simulink model "spring_calibration"  (R2016b)
settings: Solver=VariableStepAuto  StartTime=0.0  StopTime=3  RelTol=1e-3  EnableMultiTasking=on
values from neighbouring files (symbols this model uses):
  m = force(i)    [calibration.m]
  max_force = []    [calibration.m]
libraries: nesl_utility x4, fl_lib x4
settings Model: Creator=joachimdenil  LastModifiedBy=jdenil
settings DataIOCC: SaveFormat=Array
settings OptimizationCC: LifeSpan=inf
settings DebuggingCC: SFUnexpectedBacktrackingDiag=warning  SFNoUnconditionalDefaultTransitionDiag=warning  SFExecutionAtInitializationDiag=none
settings GRTTargetCC: TargetLangStandard=C89/C90 (ANSI)  GeneratePreprocessorConditionals=Disable all
settings ConfigComp: CovMetricSettings=dw  CovHtmlReporting=on  CovSaveCumulativeToWorkspaceVar=on  CovSaveSingleToWorkspaceVar=on  CovExternalEMLEnable=off

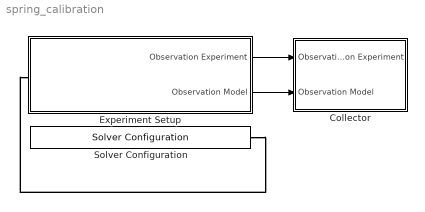
== system spring_calibration ==
  Collector : Subsystem  TreatAsAtomicUnit=on
  Experiment Setup : Subsystem
  Solver Configuration : nesl_utility/Solver Configuration  PhysicalDomain=network_engine_domain  SubClassName=solver  LeftPortType=input  RightPortType=generic  Accelerate=off  Tones=[]  Harmonics=[]  SimulateNoise=off  Profile=off  UseLocalSampling=off  EnableSwitchedLinearOptims=on  FrequencyDomain=off  UseCCode=off  RelTol=0.001  AbsTol=1e-06  MinStep=1e-09  ToWorkspace=off  RevertToSquareIcSolve=off  NumHomotopyIterations=100  PhasorMode=off  PhasorModeNumHarmonics=1  OverrideAbsTol=off  DoDC=off  ResidualTolerance=1e-09  UseLocalSolver=off  LocalSolverChoice=NE_BACKWARD_EULER_ADVANCER  LocalSolverSampleTime=0.001  DoFixedCost=off  MaxNonlinIter=3  MaxModeIter=2  LinearAlgebra=Sparse  DelaysMemoryBudget=1024  AutomaticFiltering=on  FilteringTimeConstant=0.001
  wires:
  Experiment Setup/1(Observation Experiment) -> Collector/1(Observation Experiment)
  Experiment Setup/2(Observation Model) -> Collector/2(Observation Model)
  connections:
  Solver Configuration/RConn1 -- Experiment Setup/LConn1

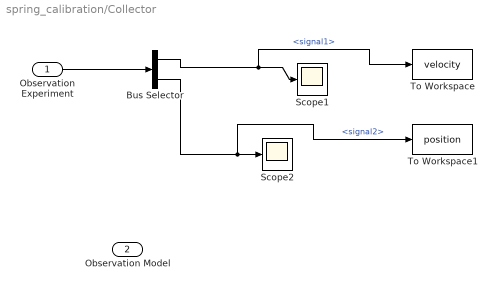
== system spring_calibration/Collector ==
  Observation Experiment : Inport
  Observation Model : Inport  Port=2
  Bus Selector : BusSelector  OutputSignals=signal1,signal2
  Scope1 : Scope
  Scope2 : Scope
  To Workspace : ToWorkspace  VariableName=velocity  SaveFormat=Timeseries  SampleTime=-1
  To Workspace1 : ToWorkspace  VariableName=position  SaveFormat=Timeseries  SampleTime=-1
  wires:
  Observation Experiment/1 -> Bus Selector/1
  Bus Selector/1 -> To Workspace/1, Scope1/1  "<signal1>"
  Bus Selector/2 -> To Workspace1/1, Scope2/1  "<signal2>"

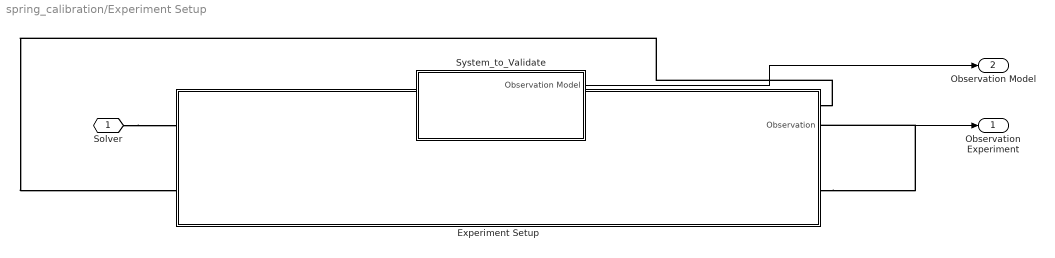
== system spring_calibration/Experiment Setup ==
  Experiment Setup : Subsystem
  System_to_Validate : Subsystem
  Solver : PMIOPort  Port=1  Side=Left
  Observation Experiment : Outport
  Observation Model : Outport  Port=2
  wires:
  System_to_Validate/1(Observation Model) -> Observation Model/1
  Experiment Setup/1(Observation) -> Observation Experiment/1
  connections:
  Experiment Setup/RConn1 -- System_to_Validate/RConn2
  System_to_Validate/RConn1 -- Experiment Setup/LConn2
  Solver/RConn1 -- Experiment Setup/LConn1

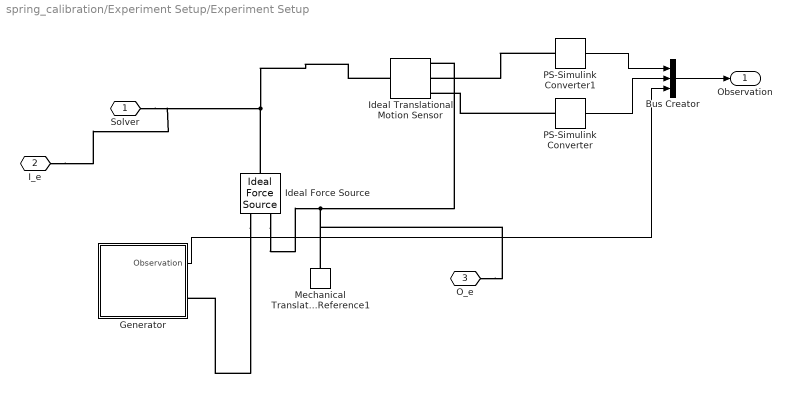
== system spring_calibration/Experiment Setup/Experiment Setup ==
  Bus Creator : BusCreator  Inputs=3
  Generator : Subsystem
  Ideal Force Source : fl_lib/Mechanical/Mechanical Sources/Ideal Force Source
  Ideal Translational Motion Sensor : fl_lib/Mechanical/Mechanical Sensors/Ideal Translational Motion Sensor  offset=0 m
  Mechanical Translational Reference1 : fl_lib/Mechanical/Translational Elements/Mechanical Translational Reference
  PS-Simulink Converter : nesl_utility/PS-Simulink Converter  PhysicalDomain=network_engine_domain  SubClassName=ps_output  LeftPortType=input  RightPortType=output  PseudoPeriodic=off  Frequencies=[]  Unit=1  AffineConversion=off
  PS-Simulink Converter1 : nesl_utility/PS-Simulink Converter  PhysicalDomain=network_engine_domain  SubClassName=ps_output  LeftPortType=input  RightPortType=output  PseudoPeriodic=off  Frequencies=[]  Unit=1  AffineConversion=off
  Solver : PMIOPort  Port=1  Side=Left
  I_e : PMIOPort  Port=2  Side=Left
  O_e : PMIOPort  Port=3  Side=Right
  Observation : Outport
  wires:
  Generator/1(Observation) -> Bus Creator/3
  PS-Simulink Converter/1 -> Bus Creator/2
  PS-Simulink Converter1/1 -> Bus Creator/1
  Bus Creator/1 -> Observation/1
  connections:
  Ideal Force Source/LConn1 -- Ideal Translational Motion Sensor/LConn1 -- I_e/RConn1 -- Solver/RConn1
  Ideal Force Source/RConn2 -- O_e/RConn1 -- Mechanical Translational Reference1/LConn1 -- Ideal Translational Motion Sensor/RConn1
  PS-Simulink Converter/LConn1 -- Ideal Translational Motion Sensor/RConn3
  PS-Simulink Converter1/LConn1 -- Ideal Translational Motion Sensor/RConn2
  Ideal Force Source/RConn1 -- Generator/RConn1

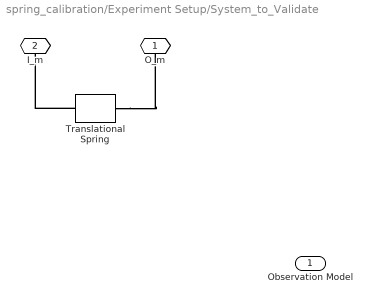
== system spring_calibration/Experiment Setup/System_to_Validate ==
  Translational Spring : fl_lib/Mechanical/Translational Elements/Translational Spring  spr_rate=k N/m  v_specify=off  v_priority=None  v=0 m/s  f_specify=off  f_priority=None  f=0 N  x_specify=on  x_priority=High  x=ic m
  O_m : PMIOPort  Port=1  Side=Right
  I_m : PMIOPort  Port=2  Side=Right
  Observation Model : Outport
  connections:
  Translational Spring/RConn1 -- O_m/RConn1
  Translational Spring/LConn1 -- I_m/RConn1

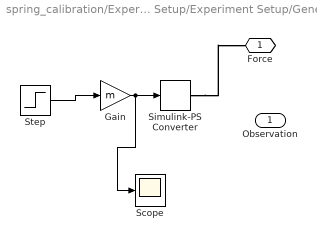
== system spring_calibration/Experiment Setup/Experiment Setup/Generator ==
  Gain : Gain  Gain=m  OutMax=max_force
  Scope : Scope
  Simulink-PS Converter : nesl_utility/Simulink-PS Converter  PhysicalDomain=network_engine_domain  SubClassName=ps_input  LeftPortType=input  RightPortType=output  PseudoPeriodic=off  Frequencies=[]  NoiseDistribution=none  NoiseParameters=[]  Unit=1  AffineConversion=off  InputFiltering=off  SimscapeFilterOrder=1  InputFilterTimeConstant=0.001  UdotUserProvided=1
  Step : Step  Time=0.1  SampleTime=0
  Force : PMIOPort  Port=1  Side=Right
  Observation : Outport
  wires:
  Gain/1 -> Scope/1, Simulink-PS Converter/1
  Step/1 -> Gain/1
  connections:
  Simulink-PS Converter/RConn1 -- Force/RConn1
